simulink model "Hinf_sim"  (Simulink 7.5)
settings: Solver=ode45  StartTime=0.0  StopTime=40  RelTol=1e-3
InitFcn:
  | start_hinf
values from neighbouring files (symbols this model uses):
  A = [-0.1778 0 0 0 0 -9.7807 -9.7807 0 0 0 0 ... (first row only)    [start_h2.m]    (also in start_hinf.m; start_lqg.m)
  Acmp = A+B*F+K*C1    [start_h2.m]    (also in start_hinf.m = A+(1/gamma^2)*E*E'*P+B*F+(eye(11)-(1/gamma^2)*Q*P)^-1*K*(C1+)
  B = [zeros(6,4) ... (first row only)    [start_h2.m]    (also in start_hinf.m; start_lqg.m)
  Bcmp = -K    [start_h2.m]    (also in start_hinf.m = -(eye(11)-(1/gamma^2)*Q*P)^-1*K)
  C1 = C    [start_h2.m]    (also in start_hinf.m)
  Ccmp = F    [start_h2.m]    (also in start_hinf.m)
  D1 = D1cap    [start_h2.m]    (also in start_hinf.m)
  E = [A(:,1),A(:,2),A(:,9)]    [start_h2.m]    (also in start_hinf.m; start_lqg.m)
  x0 = [1 0 0 0 0 -0.1 0 0 0 0 0]'    [start_h2.m]    (also in start_hinf.m; start_lqg.m)
settings Model: Creator=Prasad  LastModifiedBy=Prasad

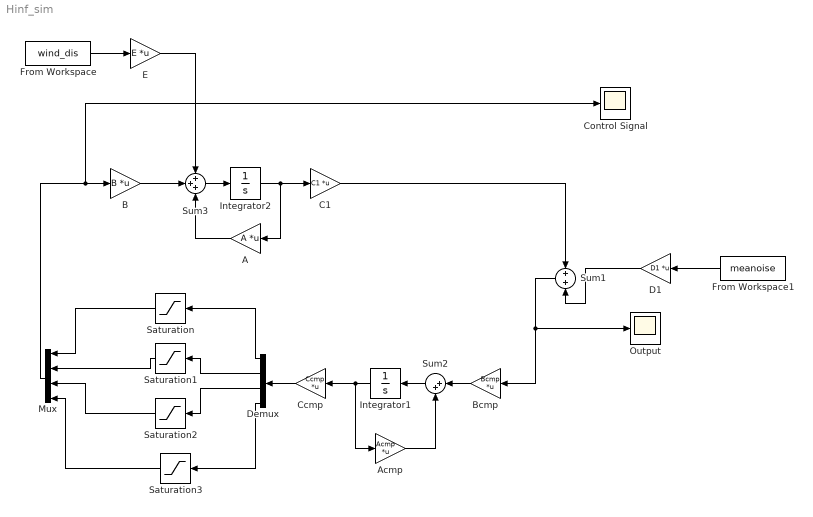
== system Hinf_sim ==
  A : Gain  Gain=A  Multiplication=Matrix(K*u)  ParameterDataType=fixdt(1, 16)  ParameterScaling=2^0  OutDataType=fixdt(1, 16)  OutScaling=2^0
  Acmp : Gain  Gain=Acmp  Multiplication=Matrix(K*u)  ParameterDataType=fixdt(1, 16)  ParameterScaling=2^0  OutDataType=fixdt(1, 16)  OutScaling=2^0
  B : Gain  Gain=B  Multiplication=Matrix(K*u)  ParameterDataType=fixdt(1, 16)  ParameterScaling=2^0  OutDataType=fixdt(1, 16)  OutScaling=2^0
  Bcmp : Gain  Gain=Bcmp  Multiplication=Matrix(K*u)  ParameterDataType=fixdt(1, 16)  ParameterScaling=2^0  OutDataType=fixdt(1, 16)  OutScaling=2^0
  C1 : Gain  Gain=C1  Multiplication=Matrix(K*u)  ParameterDataType=fixdt(1, 16)  ParameterScaling=2^0  OutDataType=fixdt(1, 16)  OutScaling=2^0
  Ccmp : Gain  Gain=Ccmp  Multiplication=Matrix(K*u)  ParameterDataType=fixdt(1, 16)  ParameterScaling=2^0  OutDataType=fixdt(1, 16)  OutScaling=2^0
  Control Signal : Scope
      settings: TimeRange=10  YMin=-0.4  YMax=1.2
  D1 : Gain  Gain=D1  Multiplication=Matrix(K*u)  ParameterDataType=fixdt(1, 16)  ParameterScaling=2^0  OutDataType=fixdt(1, 16)  OutScaling=2^0
  Demux : Demux
  E : Gain  Gain=E  Multiplication=Matrix(K*u)  ParameterDataType=fixdt(1, 16)  ParameterScaling=2^0  OutDataType=fixdt(1, 16)  OutScaling=2^0
  From Workspace : FromWorkspace  VariableName=wind_dis  SampleTime=0  OutputAfterFinalValue=Holding final value
  From Workspace1 : FromWorkspace  VariableName=meanoise  SampleTime=0  OutputAfterFinalValue=Holding final value
  Integrator1 : Integrator
  Integrator2 : Integrator  InitialCondition=x0
  Mux : Mux
  Output : Scope
      settings: TimeRange=10  YMin=-0.4  YMax=1.2
  Saturation : Saturate  UpperLimit=0.35  LowerLimit=-0.35  OutDataType=fixdt(1, 16)  OutScaling=2^0
  Saturation1 : Saturate  UpperLimit=0.35  LowerLimit=-0.35  OutDataType=fixdt(1, 16)  OutScaling=2^0
  Saturation2 : Saturate  UpperLimit=0.12  LowerLimit=-0.12  OutDataType=fixdt(1, 16)  OutScaling=2^0
  Saturation3 : Saturate  UpperLimit=0.4  LowerLimit=-0.4  OutDataType=fixdt(1, 16)  OutScaling=2^0
  Sum1 : Sum  OutDataType=fixdt(1, 16)  OutScaling=2^0
  Sum2 : Sum  Inputs=|++  OutDataType=fixdt(1, 16)  OutScaling=2^0
  Sum3 : Sum  Inputs=+++  OutDataType=fixdt(1, 16)  OutScaling=2^0
  wires:
  Integrator1/1 -> Ccmp/1, Acmp/1
  Sum2/1 -> Integrator1/1
  Acmp/1 -> Sum2/2
  Bcmp/1 -> Sum2/1
  Demux/1 -> Saturation/1
  Demux/2 -> Saturation1/1
  Demux/3 -> Saturation2/1
  Demux/4 -> Saturation3/1
  Saturation/1 -> Mux/1
  Saturation1/1 -> Mux/2
  Saturation2/1 -> Mux/3
  Saturation3/1 -> Mux/4
  Ccmp/1 -> Demux/1
  Mux/1 -> B/1, Control Signal/1
  Sum3/1 -> Integrator2/1
  Integrator2/1 -> C1/1, A/1
  E/1 -> Sum3/1
  A/1 -> Sum3/3
  From Workspace/1 -> E/1
  B/1 -> Sum3/2
  C1/1 -> Sum1/1
  Sum1/1 -> Bcmp/1, Output/1
  D1/1 -> Sum1/2
  From Workspace1/1 -> D1/1
